simulink model "PlantModel_sim_2020"  (R2020b)
settings: Solver=ode4  StartTime=0.0  StopTime=10.0  FixedStep=0.05  RelTol=1e-3
libraries: MBDLib_2020 x4
settings Model: Creator=005274  LastModifiedBy=005274

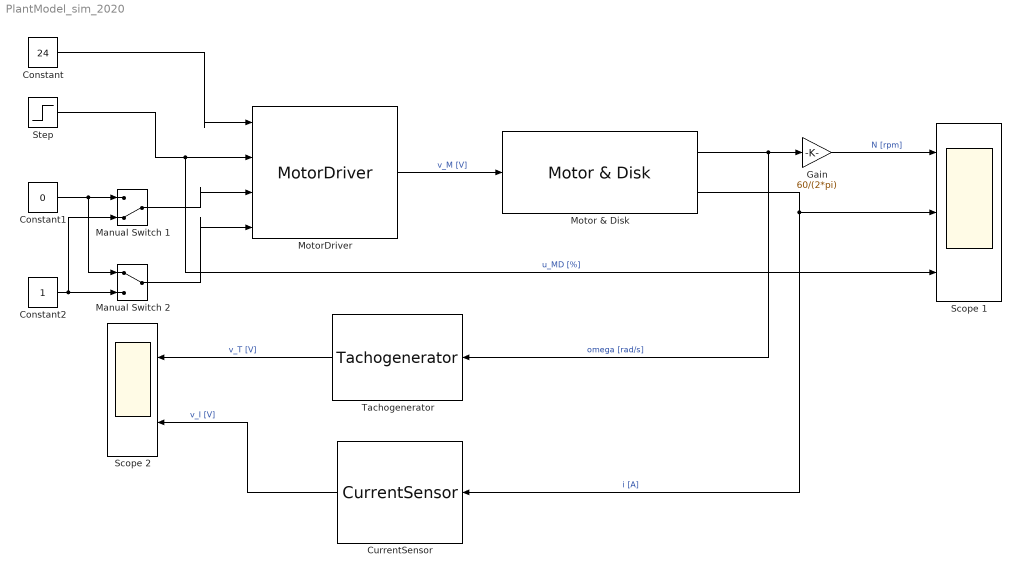
== system PlantModel_sim_2020 ==
  Constant : Constant  Value=24
  Constant1 : Constant  Value=0
  Constant2 : Constant
  "CurrentSensor " : MBDLib_2020/Sensor/CurrentSensor
      settings: SourceProductName=MBDLibrary
  Gain : Gain  Gain=60/(2*pi)
  "Manual Switch 1 " : ManualSwitch  CurrentSetting=0
  Manual Switch 2 : ManualSwitch
  "Motor & Disk " : MBDLib_2020/Plant/Motor & Disk  R=5.7  L=0.2  J_M=1.1e-4  J_I=1.3e-3  D=6.0e-5  K_tau=7.2e-2  K_e=7.2e-2
      settings: SourceProductName=MBDLibrary
  "MotorDriver " : MBDLib_2020/Actuator/MotorDriver
      settings: SourceProductName=MBDLibrary
  Scope 1 : Scope  NumInputPorts=3
  Scope 2 : Scope  NumInputPorts=2
  Step : Step  After=100  SampleTime=0
  "Tachogenerator " : MBDLib_2020/Sensor/Tachogenerator
      settings: SourceProductName=MBDLibrary
  wires:
  "MotorDriver "/1 -> "Motor & Disk "/1  "v_M [V]"
  Step/1 -> Scope 1/3, "MotorDriver "/2  "u_MD [%]"
  Constant/1 -> "MotorDriver "/1
  Constant2/1 -> "Manual Switch 1 "/2, Manual Switch 2/2
  Constant1/1 -> Manual Switch 2/1, "Manual Switch 1 "/1
  "Manual Switch 1 "/1 -> "MotorDriver "/3
  Manual Switch 2/1 -> "MotorDriver "/4
  "Motor & Disk "/1 -> "Tachogenerator "/1, Gain/1  "omega [rad/s]"
  "Motor & Disk "/2 -> "CurrentSensor "/1, Scope 1/2  "i [A]"
  Gain/1 -> Scope 1/1  "N [rpm]"
  "CurrentSensor "/1 -> Scope 2/2  "v_I [V]"
  "Tachogenerator "/1 -> Scope 2/1  "v_T [V]"
